simulink model "task11lab1"  (R2022b)
settings: Solver=VariableStepAuto  StartTime=0.0  StopTime=10.0  RelTol=1e-3
settings Model: Creator=af063  LastModifiedBy=af063

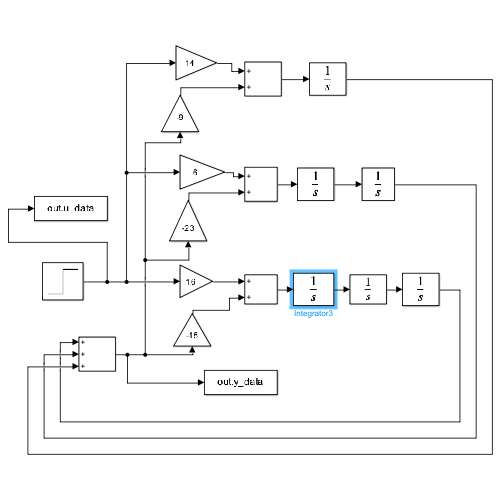
[thumbnail: Simulink's stored preview of the top-level diagram]
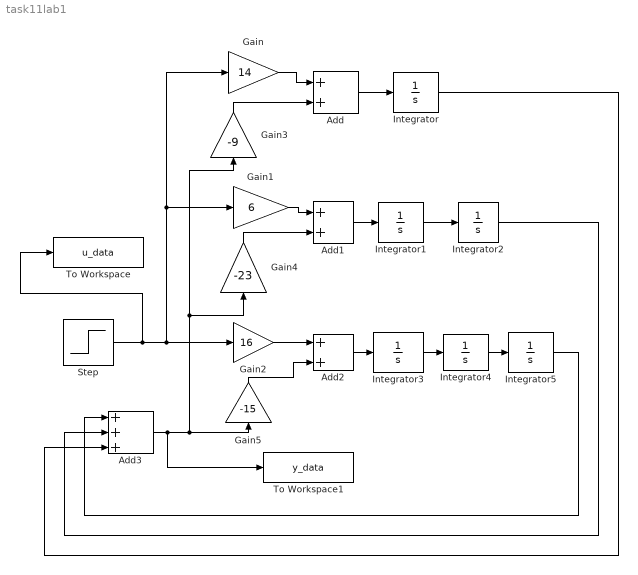
== system task11lab1 ==
  Add : Sum
  Add1 : Sum
  Add2 : Sum
  Add3 : Sum  Inputs=+++
  Gain : Gain  Gain=14
  Gain1 : Gain  Gain=6
  Gain2 : Gain  Gain=16
  Gain3 : Gain  Gain=-9
  Gain4 : Gain  Gain=-23
  Gain5 : Gain  Gain=-15
  Integrator : Integrator  InitialCondition=1
  Integrator1 : Integrator  InitialCondition=9.1
  Integrator2 : Integrator
  Integrator3 : Integrator  InitialCondition=24.4
  Integrator4 : Integrator
  Integrator5 : Integrator
  Step : Step  Time=0  SampleTime=0
  To Workspace : ToWorkspace  VariableName=u_data  SampleTime=-1
  To Workspace1 : ToWorkspace  VariableName=y_data  SampleTime=-1
  wires:
  Step/1 -> To Workspace/1, Gain2/1, Gain/1, Gain1/1
  Gain/1 -> Add/1
  Gain3/1 -> Add/2
  Gain1/1 -> Add1/1
  Gain4/1 -> Add1/2
  Gain2/1 -> Add2/1
  Gain5/1 -> Add2/2
  Add/1 -> Integrator/1
  Integrator/1 -> Add3/3
  Add1/1 -> Integrator1/1
  Integrator1/1 -> Integrator2/1
  Integrator2/1 -> Add3/2
  Add3/1 -> To Workspace1/1, Gain5/1, Gain4/1, Gain3/1
  Add2/1 -> Integrator3/1
  Integrator3/1 -> Integrator4/1
  Integrator4/1 -> Integrator5/1
  Integrator5/1 -> Add3/1
